simulink model "Simscape_Actuated_Robot"  (R2025b)
settings: Solver=ode45  StartTime=0.0  StopTime=20  RelTol=1e-3
InitFcn:
  | run("init.m");
values from neighbouring files (symbols this model uses):
  q0_guess = [pi/3; -pi/6; pi/3]    [init.m]
  q_init = [pi/6,-pi/3, 0,pi/6,-pi/3,0]    [init.m]
  Ts = 1e-3    (= 0.001)    [init.m]
undefined symbols (not defined in the file or in its folder): robot_params, X, Y, Z
libraries: sm_lib x48, nesl_utility x48
(part 3 of 3)

== matlab function Simscape_Actuated_Robot/Subsystem/MATLAB Function8 ==
  settings: updateMethod=DISCRETE
  data: q1_ginocchio input; l output; q2_anca input; q3_torso input; theta output; I_y output; theta_dot output
function [l, theta, I_y, theta_dot] = calculate_equivalent_pendulum_v3(q1_ginocchio, q2_anca, q3_torso)
    persistent theta_prev
    if isempty(theta_prev), theta_prev = 0; end
    dt = 0.001;

    m1=1.2; m2=5.3; m3=60.0;
    l1=0.45; l2=0.45; l3=0.35;

    phi_shank = q1_ginocchio - q2_anca + q3_torso;
    phi_thigh = q3_torso - q2_anca;

    x1 = (l1/2)*sin(phi_shank);              y1 = (l1/2)*cos(phi_shank);
    xk = l1*sin(phi_shank);                  yk = l1*cos(phi_shank);
    x2 = xk + (l2/2)*sin(phi_thigh);         y2 = yk + (l2/2)*cos(phi_thigh);
    xh = xk + l2*sin(phi_thigh);             yh = yk + l2*cos(phi_thigh);
    x3 = xh + (l3/2)*sin(q3_torso);          y3 = yh + (l3/2)*cos(q3_torso);

    m_tot = m1+m2+m3;
    SC = (m1*x1 + m2*x2 + m3*x3) / m_tot;
    ZC = (m1*y1 + m2*y2 + m3*y3) / m_tot;

    l = sqrt(SC^2 + ZC^2);
    if l < 0.1, l = 0.1; end

    theta = atan2(SC, ZC);

    % Unwrap per evitare i falsi picchi di theta_dot
    delta_theta = theta - theta_prev;
    delta_theta = atan2(sin(delta_theta), cos(delta_theta));
    theta_dot = delta_theta / dt;
    theta_prev = theta;

    I_y = (1/3) * m_tot * l^2;
end

== matlab function Simscape_Actuated_Robot/Subsystem/MATLAB Function9 ==
  data: X input; U output; X_ref input; l input; I_y input
function U = TV_LQR_Controller(X, X_ref, l, I_y)
    % X: Stato attuale [s; theta; phi; s_dot; theta_dot; phi_dot] (6x1)
    % X_ref: Stato target desiderato [s_ref; theta_ref; phi_ref; 0; 0; 0] (6x1)
    % l: Lunghezza attuale del pendolo equivalente [m]
    % I_y: Inerzia attuale del corpo superiore [kg*m^2]
    
    % Per usare la funzione lqr() di MATLAB all'interno di Simulink, 
    % dobbiamo dichiararla come estrinseca.
    coder.extrinsic('lqr');
    if l < 0.1
        l = 0.1;
    end
    if I_y < 1e-3
        I_y = 1e-3;
    end
    % 1. Richiamo Parametri Fisici
    m_w = 3.5;       % Massa ruota
    I_w = 0.1;       % Inerzia ruota
    r   = 0.127;     % Raggio ruota
    d   = 0.63;      % Distanza ruote
    m_b = 73.0;      % Massa corpo superiore
    I_z = 3.3;       % Inerzia torso asse z
    g   = 9.81;      % Gravità
    
    % 2. Calcolo dei Coefficienti della Dinamica (Eq. 14)
    % Denominatore comune per a1, a2, b1, b2
    D = 2*I_w*(I_y + m_b*l^2) + (2*l^2*m_b*m_w + I_y*(m_b + 2*m_w)*r^2);
    
    a1 = -(g * l^2 * m_b^2 * r^2) / D;
    a2 =  (g * l * m_b * (2*I_w + (m_b + 2*m_w)*r^2)) / D;
    
    b1 =  (r * (I_y + l*m_b*(l + r))) / D;
    b2 = -(2*I_w + r*(l*m_b + (m_b + 2*m_w)*r)) / D;
    
    % Coefficiente disaccoppiato per lo steering (imbardata)
    b3 =  (d * r) / (2*I_z*r^2 + d^2*(I_w + m_w*r^2));
    
    % 3. Costruzione Matrici di Stato A(l) e Input B(l) (Eq. 12, Eq. 13)
    A = zeros(6, 6);
    A(1, 4) = 1; 
    A(2, 5) = 1; 
    A(3, 6) = 1;
    A(4, 2) = a1;
    A(5, 2) = a2;
    
    B = zeros(6, 2);
    B(4, 1) = b1;  B(4, 2) = b1;
    B(5, 1) = b2;  B(5, 2) = b2;
    B(6, 1) = b3;  B(6, 2) = -b3;
    
    % 4. Definizione Matrici di Peso Q e R (Tuning LQR)
    % Questi valori determinano l'aggressività del controllore. 
    % Possono essere trasformati in input del blocco per un tuning rapido.
    % 4. Definizione Matrici di Peso Q e R (Tuning Soft)
    % Pesi drasticamente ridotti per evitare instabilità con il ritardo discreto
% Aumenta il peso sugli angoli (q1, q2) per evitare che saturino
%X = [s, θ, φ, ṡ, θ̇, φ̇]
    Q = diag([50, 50, 100, 50, 10, 1]);
    R = diag([1, 1]) * 0.5;         % uso coppie piu abbasso piu accelera
    
    % 5. Risoluzione LQR e Calcolo Input
    % Inizializza K per la Code Generation di Simulink
    K = zeros(2, 6); 
    
    % Calcola la matrice dei guadagni ottimali K
    K = lqr(A, B, Q, R);
    
    % Errore di stato (tilde_X)
    X_tilde = X - X_ref;
    
    % Legge di controllo finale (Eq. 16): U = [tau_l; tau_r]
    U = -K * X_tilde; 
end

== matlab function Simscape_Actuated_Robot/MATLAB Function2 ==
  settings: updateMethod=DISCRETE  sampleTime=0.1
  data: h_des input; q_des output; robot_params parameter; q0_guess parameter
function q_des = fcn(h_des, robot_params, q0_guess)
    % 1. Pre-allocazione per dire a Simulink che uscirà un vettore 3x1
    q_des = zeros(3,1);
    
    % 2. Dichiara la TUA funzione esterna come estrinseca (non fsolve)
    coder.extrinsic('calcola_target_cinematici');
    
    % 3. Inizializza la variabile temporanea per aiutare il Coder con i tipi
    q_des_calc = zeros(3,1);
    
    % 4. Richiama la funzione (il calcolo viene "appaltato" a MATLAB)
    q_des_calc = calcola_target_cinematici(h_des, robot_params, q0_guess);
    
    % 5. Assegnazione sicura all'uscita
    if ~isempty(q_des_calc)
        q_des = q_des_calc;
    end
end

== matlab function Simscape_Actuated_Robot/Subsystem1/MATLAB Function9 ==
  data: X input; U output; X_ref input; l input; I_y input
function U = TV_LQR_Controller(X, X_ref, l, I_y)
    % X: Stato attuale [s; theta; phi; s_dot; theta_dot; phi_dot] (6x1)
    % X_ref: Stato target desiderato [s_ref; theta_ref; phi_ref; 0; 0; 0] (6x1)
    % l: Lunghezza attuale del pendolo equivalente [m]
    % I_y: Inerzia attuale del corpo superiore [kg*m^2]
    
    % Per usare la funzione lqr() di MATLAB all'interno di Simulink, 
    % dobbiamo dichiararla come estrinseca.
    coder.extrinsic('lqr');
    if l < 0.1
        l = 0.1;
    end
    if I_y < 1e-3
        I_y = 1e-3;
    end
    % 1. Richiamo Parametri Fisici
    m_w = 3.5;       % Massa ruota
    I_w = 0.1;       % Inerzia ruota
    r   = 0.127;     % Raggio ruota
    d   = 0.63;      % Distanza ruote
    m_b = 73.0;      % Massa corpo superiore
    I_z = 3.3;       % Inerzia torso asse z
    g   = 9.81;      % Gravità
    
    % 2. Calcolo dei Coefficienti della Dinamica (Eq. 14)
    % Denominatore comune per a1, a2, b1, b2
    D = 2*I_w*(I_y + m_b*l^2) + (2*l^2*m_b*m_w + I_y*(m_b + 2*m_w)*r^2);
    
    a1 = -(g * l^2 * m_b^2 * r^2) / D;
    a2 =  (g * l * m_b * (2*I_w + (m_b + 2*m_w)*r^2)) / D;
    
    b1 =  (r * (I_y + l*m_b*(l + r))) / D;
    b2 = -(2*I_w + r*(l*m_b + (m_b + 2*m_w)*r)) / D;
    
    % Coefficiente disaccoppiato per lo steering (imbardata)
    b3 =  (d * r) / (2*I_z*r^2 + d^2*(I_w + m_w*r^2));
    
    % 3. Costruzione Matrici di Stato A(l) e Input B(l) (Eq. 12, Eq. 13)
    A = zeros(6, 6);
    A(1, 4) = 1; 
    A(2, 5) = 1; 
    A(3, 6) = 1;
    A(4, 2) = a1;
    A(5, 2) = a2;
    
    B = zeros(6, 2);
    B(4, 1) = b1;  B(4, 2) = b1;
    B(5, 1) = b2;  B(5, 2) = b2;
    B(6, 1) = b3;  B(6, 2) = -b3;
    
    % 4. Definizione Matrici di Peso Q e R (Tuning LQR)
    % Questi valori determinano l'aggressività del controllore. 
    % Possono essere trasformati in input del blocco per un tuning rapido.
    % 4. Definizione Matrici di Peso Q e R (Tuning Soft)
    % Pesi drasticamente ridotti per evitare instabilità con il ritardo discreto
% Aumenta il peso sugli angoli (q1, q2) per evitare che saturino
%X = [s, θ, φ, ṡ, θ̇, φ̇]
    Q = diag([50, 50, 100, 50, 10, 1]);
    R = diag([1, 1]) * 0.5;         % uso coppie piu abbasso piu accelera
    
    % 5. Risoluzione LQR e Calcolo Input
    % Inizializza K per la Code Generation di Simulink
    K = zeros(2, 6); 
    
    % Calcola la matrice dei guadagni ottimali K
    K = lqr(A, B, Q, R);
    
    % Errore di stato (tilde_X)
    X_tilde = X - X_ref;
    
    % Legge di controllo finale (Eq. 16): U = [tau_l; tau_r]
    U = -K * X_tilde; 
end

== matlab function Simscape_Actuated_Robot/Subsystem1/MATLAB Function ==
  data: Delta_s_des input; tau_leg output; F_z_mpc input; q1_ginocchio input; q2_anca input
function tau_leg = VMC_Task_Space_Controller(Delta_s_des, F_z_mpc, q1_ginocchio, q2_anca)
    tau_leg = zeros(2, 1);
    l = 0.45; m_tot = 73.0; g = 9.81;
    % --- Ginocchio: gestisce F_z (invariato) ---
    J_z_knee = -l * sin(q1_ginocchio / 2);
    if abs(J_z_knee) < 0.05, J_z_knee = -0.05 * sign(q1_ginocchio + 1e-6); end
    F_z_totale = F_z_mpc + (m_tot * g);
    tau_k = J_z_knee * F_z_totale;
    % --- Anca: PD verso un target proporzionale a Delta_s_des ---
    l_pendolo = 0.85;   % lunghezza approssimata del pendolo equivalente
    q2_anca_target = -Delta_s_des / l_pendolo;
    Kp_h = 400;
    Kd_h = 40;
    tau_h = -Kp_h * (q2_anca - q2_anca_target) - Kd_h * (0);  % termine derivativo omesso per ora
    tau_leg = [tau_k; tau_h];
end

== matlab function Simscape_Actuated_Robot/Subsystem1/MATLAB Function7 ==
  settings: updateMethod=DISCRETE
  data: tau_leg output; F_z_mpc input; q1_ginocchio input; q2_anca input; q3_torso input
function tau_leg  = VMC_Task_Space_Controller(F_z_mpc, q1_ginocchio, q2_anca, q3_torso)

% =========================================================================

% VMC CORRETTO - Ripartizione pulita delle competenze della GAMBA:

%   GINOCCHIO -> altezza z          (canale verticale)

%   ANCA      -> beccheggio torso q3 (stabilizzazione, anello prima mancante)

% Lo spostamento ORIZZONTALE del CoM NON e' piu' gestito qui: e' compito

% della ruota (TV-LQR). Cosi' sparisce il conflitto che destabilizzava l'MPC.

%

% Delta_s_des, s_actual, s_dot_actual, dq2_anca restano solo per compatibilita'

% di cablaggio (non sono piu' usati per il controllo dell'anca).

% =========================================================================
 
    % --- Uscite inizializzate (necessario per code generation) ---

    tau_leg   = zeros(2,1);

    SC_out    = 0.0;

    J_hip_out = 0.0;
 
    % --- Parametri fisici ---

    l1 = 0.45; l2 = 0.45;

    z_des = 0.6;          % altezza di equilibrio (asse ruota -> anca) [m]

    dt    = 0.001;        % deve coincidere col passo fisso del solutore
 
    % --- Stima derivate via differenza finita (persistenti) ---

    persistent q3_prev z_prev

    if isempty(q3_prev), q3_prev = q3_torso; end
 
    % Cinematica utile

    phi_shank = q1_ginocchio - q2_anca + q3_torso;

    phi_thigh = q3_torso - q2_anca;

    z_actual  = l1*cos(phi_shank) + l2*cos(phi_thigh);
 
    if isempty(z_prev), z_prev = z_actual; end
 
    dq3   = (q3_torso - q3_prev)/dt;   q3_prev = q3_torso;

    z_dot = (z_actual - z_prev)/dt;    z_prev  = z_actual;
 
    % --- CoM: solo per monitoraggio/uscite ---

    coder.extrinsic('calc_com_jacobian');

    J_SC = zeros(1,2); J_ZC = zeros(1,2); SC = 0.0; ZC = 0.0;

    [J_SC, J_ZC, SC, ZC] = calc_com_jacobian(q1_ginocchio, q2_anca, q3_torso);

    SC_out    = SC;

    J_hip_out = J_SC(2);
 
    % --- Compensazione di gravita' dalla dinamica VERA G(q) ---

    % (sostituisce il vecchio Jacobiano del ginocchio "clampato", instabile

    %  a gamba dritta). G non dipende da dq, quindi passo dq = 0.

    coder.extrinsic('calc_dynamics');

    q_full  = [q1_ginocchio; 0; q2_anca; q3_torso];   % ordine [q1;qw;q2;q3]

    M   = zeros(4,4); CdQ = zeros(4,1); G = zeros(4,1);

    [M, CdQ, G] = calc_dynamics(q_full, zeros(4,1));

    tau_k_grav = G(1);   % coppia statica ginocchio

    tau_h_grav = G(3);   % coppia statica anca
 
    % =====================================================================

    % (1) GINOCCHIO  ->  controllo di ALTEZZA

    % =====================================================================

    Kp_z = 4000; Kd_z = 300;               % PD altezza (DA TARARE)

    Jz_knee = -l1*sin(phi_shank);          % dz/dq1

    if abs(Jz_knee) < 0.05                  % vicino a gamba dritta: autorita' ~0

        Jz_knee = 0.05*sign(Jz_knee + 1e-9);

    end

    F_z_cmd = Kp_z*(z_des - z_actual) - Kd_z*z_dot + F_z_mpc;  % forza vert. extra

    tau_k   = tau_k_grav + Jz_knee * F_z_cmd;
 
    % =====================================================================

    % (2) ANCA  ->  stabilizza il BECCHEGGIO del torso  q3 -> 0

    % =====================================================================

    Kp_t = 800; Kd_t = 80;                 % PD torso (DA TARARE)

    % SEGNO: parti con -(Kp*q3 + Kd*dq3). Se in simulazione il torso DIVERGE

    %        invece di raddrizzarsi, INVERTI il segno del termine PD.

    tau_h = tau_h_grav - (Kp_t*q3_torso + Kd_t*dq3);
 
    tau_leg = [tau_k; tau_h];

end

== matlab function Simscape_Actuated_Robot/Subsystem1/MATLAB Function8 ==
  settings: updateMethod=DISCRETE
  data: q1_ginocchio input; l output; q2_anca input; q3_torso input; theta output; I_y output; theta_dot output
function [l, theta, I_y, theta_dot] = calculate_equivalent_pendulum_v3(q1_ginocchio, q2_anca, q3_torso)
    persistent theta_prev
    if isempty(theta_prev), theta_prev = 0; end
    dt = 0.001;

    m1=1.2; m2=5.3; m3=60.0;
    l1=0.45; l2=0.45; l3=0.35;

    phi_shank = q1_ginocchio - q2_anca + q3_torso;
    phi_thigh = q3_torso - q2_anca;

    x1 = (l1/2)*sin(phi_shank);              y1 = (l1/2)*cos(phi_shank);
    xk = l1*sin(phi_shank);                  yk = l1*cos(phi_shank);
    x2 = xk + (l2/2)*sin(phi_thigh);         y2 = yk + (l2/2)*cos(phi_thigh);
    xh = xk + l2*sin(phi_thigh);             yh = yk + l2*cos(phi_thigh);
    x3 = xh + (l3/2)*sin(q3_torso);          y3 = yh + (l3/2)*cos(q3_torso);

    m_tot = m1+m2+m3;
    SC = (m1*x1 + m2*x2 + m3*x3) / m_tot;
    ZC = (m1*y1 + m2*y2 + m3*y3) / m_tot;

    l = sqrt(SC^2 + ZC^2);
    if l < 0.1, l = 0.1; end

    theta = atan2(SC, ZC);

    % Unwrap per evitare i falsi picchi di theta_dot
    delta_theta = theta - theta_prev;
    delta_theta = atan2(sin(delta_theta), cos(delta_theta));
    theta_dot = delta_theta / dt;
    theta_prev = theta;

    I_y = (1/3) * m_tot * l^2;
end

== matlab function Simscape_Actuated_Robot/MATLAB Function1 ==
  data: alpha output; CoM_p input; wx output; center_p input; CoM_v input; center_v input
function [alpha, wx] = fcn(CoM_p, center_p, CoM_v, center_v)
    % 1. Vettore posizione relativa (r) e velocità relativa (r_dot)
    r = CoM_p - center_p;
    r_dot = CoM_v - center_v;
    
    % 2. Estrazione delle componenti vettoriali per leggibilità (X=1, Y=2, Z=3)
    rx = r(1); 
    ry = r(2); 
    rz = r(3);
    
    rx_dot = r_dot(1); 
    ry_dot = r_dot(2); 
    rz_dot = r_dot(3);
    
    % 3. Calcolo del modulo (norma) del vettore r e la sua potenza al cubo
    norm_r = sqrt(rx^2 + ry^2 + rz^2);
    
    % 4. Calcolo del termine (rx*rx_dot + ry*ry_dot + rz*rz_dot) 
    % che corrisponde al prodotto scalare (dot product)
    dot_r = rx*rx_dot + ry*ry_dot + rz*rz_dot;
    
    % 5. Derivata dell'argomento della funzione: d/dt (rx / ||r||)
    d_arg = (rx_dot / norm_r) - (rx * dot_r) / norm_r.^3;
    
    % 6. Calcolo finale applicando la derivata dell'arcoseno per ottenere wx (ovvero alpha_dot)
    wx = (1 / sqrt(1 - (rx / norm_r)^2)) * d_arg;
    alpha = asin(rx./norm_r);

end

== matlab function Simscape_Actuated_Robot/Joint_Controllers R ==
  data: tau_hip output; q_des input; tau_knee output; q input; dq input
function [tau_hip, tau_knee] = PD_Joints(q_des, q, dq)

    Kp_j = 800;%800; 
    Kd_j = 50;%50;  
    
    e2 = q_des(1) - q(1);
    de2 = 0 - dq(1);
    tau_hip = Kp_j * e2 + Kd_j * de2;
    
    e3 = q_des(2) - q(2);
    de3 = 0 - dq(2);
    tau_knee = Kp_j * e3 + Kd_j * de3;

== matlab function Simscape_Actuated_Robot/Joint_Controllers L ==
  data: tau_hip output; q_des input; tau_knee output; q input; dq input
function [tau_hip, tau_knee] = PD_Joints(q_des, q, dq)

    Kp_j = 800;%800; 
    Kd_j = 50;%50;  
    
    e2 = q_des(1) - q(1);
    de2 = 0 - dq(1);
    tau_hip = Kp_j * e2 + Kd_j * de2;
    
    e3 = q_des(2) - q(2);
    de3 = 0 - dq(2);
    tau_knee = Kp_j * e3 + Kd_j * de3;

== matlab function Simscape_Actuated_Robot/Subsystem/MATLAB Function ==
  data: Delta_s_des input; tau_leg output; F_z_mpc input; q1_ginocchio input; q2_anca input
function tau_leg = VMC_Task_Space_Controller(Delta_s_des, F_z_mpc, q1_ginocchio, q2_anca)
    tau_leg = zeros(2, 1);
    l = 0.45; m_tot = 73.0; g = 9.81;
    % --- Ginocchio: gestisce F_z (invariato) ---
    J_z_knee = -l * sin(q1_ginocchio / 2);
    if abs(J_z_knee) < 0.05, J_z_knee = -0.05 * sign(q1_ginocchio + 1e-6); end
    F_z_totale = F_z_mpc + (m_tot * g);
    tau_k = J_z_knee * F_z_totale;
    % --- Anca: PD verso un target proporzionale a Delta_s_des ---
    l_pendolo = 0.85;   % lunghezza approssimata del pendolo equivalente
    q2_anca_target = -Delta_s_des / l_pendolo;
    Kp_h = 400;
    Kd_h = 40;
    tau_h = -Kp_h * (q2_anca - q2_anca_target) - Kd_h * (0);  % termine derivativo omesso per ora
    tau_leg = [tau_k; tau_h];
end

== matlab function Simscape_Actuated_Robot/MATLAB Function5 ==
  data: x_current input; Delta_s output; x_desired input; F_z output
function [Delta_s, F_z] = MPC_Custom_QP(x_current, x_desired)
    % quadprog non è supportato nativamente per la code generation C
    coder.extrinsic('quadprog');
    coder.extrinsic('optimoptions');

    %% 1. Parametri e Discretizzazione
    m_b = 73.0; 
    g = 9.81;    
    
    h = x_current(3); 
    if h < 0.1
        h = 0.6;
    end
    
    dt = 0.01; 
    N = 40;     
    
    A_c = zeros(5,5);
    A_c(1,2) = 1;
    A_c(3,4) = 1;
    A_c(2,5) = g / h; 
    
    B_c = zeros(5,2);
    B_c(4,2) = 1 / m_b;
    B_c(5,1) = 1;
    
    A_d = eye(5) + A_c * dt;
    B_d = B_c * dt;

    %% 2. Pesi della Funzione di Costo
    %x = [s, ṡ, z, ż, Δs]
    S = diag([1, 1, 500, 50, 1]);
    W = diag([1, 0.01]);

    %% 3. Condensazione (Srotolamento) 
    nx = 5; nu = 2;
    P_x = zeros(nx*N, nx);
    P_u = zeros(nx*N, nu*N);

    A_power = eye(nx);
    for i = 1:N
        A_power = A_power * A_d;
        P_x((i-1)*nx+1 : i*nx, :) = A_power;
        for j = 1:i
            P_u((i-1)*nx+1 : i*nx, (j-1)*nu+1 : j*nu) = (A_d^(i-j)) * B_d;
        end
    end

    S_bar = kron(eye(N), S);
    W_bar = kron(eye(N), W);

    H = 2 * (P_u' * S_bar * P_u + W_bar);
    H = (H + H') / 2; % Garantisce simmetria perfetta
    
    X_ref = repmat(x_desired, N, 1);
    f = 2 * P_u' * S_bar * (P_x * x_current - X_ref);

    %% 4. Vincoli Fisici
    F_min = -1500; % Permette di frenare!
    F_max = 1500;
    
    LB = zeros(nu*N, 1);
    UB = zeros(nu*N, 1);
    
    for i = 1:N
        LB((i-1)*nu+1) = -0.20;   % era -2.0

        UB((i-1)*nu+1) =  0.20;   % era  2.0
 
        
        LB((i-1)*nu+2) = F_min; 
        UB((i-1)*nu+2) = F_max;
    end

    %% 5. Risoluzione QP (CORRETTA)
    % Pre-allocazione per Simulink Coder
    U_opt_calc = zeros(nu*N, 1);
    fval = 0.0;
    exitflag = 0.0;
    
    % Algoritmo robusto di default
    options = optimoptions('quadprog', 'Display', 'off');
    
    % LA CORREZIONE: Aggiunto "fval" per non sballare "exitflag"!
    [U_opt_calc, fval, exitflag] = quadprog(H, f, [], [], [], [], LB, UB, [], options);

    if exitflag > 0
        U_opt = U_opt_calc;
    else
        % Se fallisce davvero, eroga 0 extra, ma il VMC ci terrà in piedi col peso base
        U_opt = zeros(nu*N, 1);
    end

    %% 6. Estrazione Input Ottimo
    Delta_s_dot_opt = U_opt(1);
    F_z = U_opt(2); % FINALMENTE SARA' DIVERSO DA ZERO!

    Delta_s = x_current(5) + Delta_s_dot_opt * dt;
end
